simulink model "testALU"  (R2025b)
settings: Solver=VariableStepAuto  StartTime=0.0  StopTime=10.0  RelTol=1e-3
settings Model: Creator=cyber  LastModifiedBy=cyber

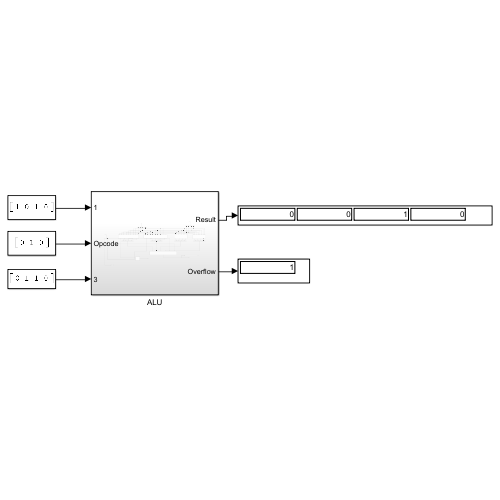
[thumbnail: Simulink's stored preview of the top-level diagram]
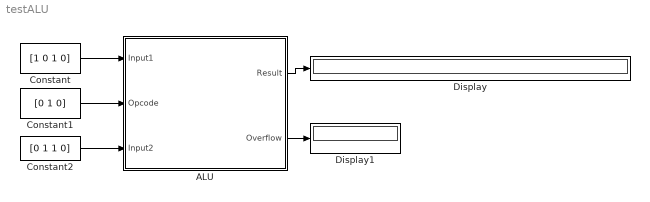
== system testALU ==
  ALU : Subsystem
  Constant : Constant  Value=[1 0 1 0]
  Constant1 : Constant  Value=[0 1 0]
  Constant2 : Constant  Value=[0 1 1 0]
  Display : Display
  Display1 : Display
  wires:
  Constant/1 -> ALU/1(Input1)
  Constant1/1 -> ALU/2(Opcode)
  Constant2/1 -> ALU/3(Input2)
  ALU/1(Result) -> Display/1
  ALU/2(Overflow) -> Display1/1

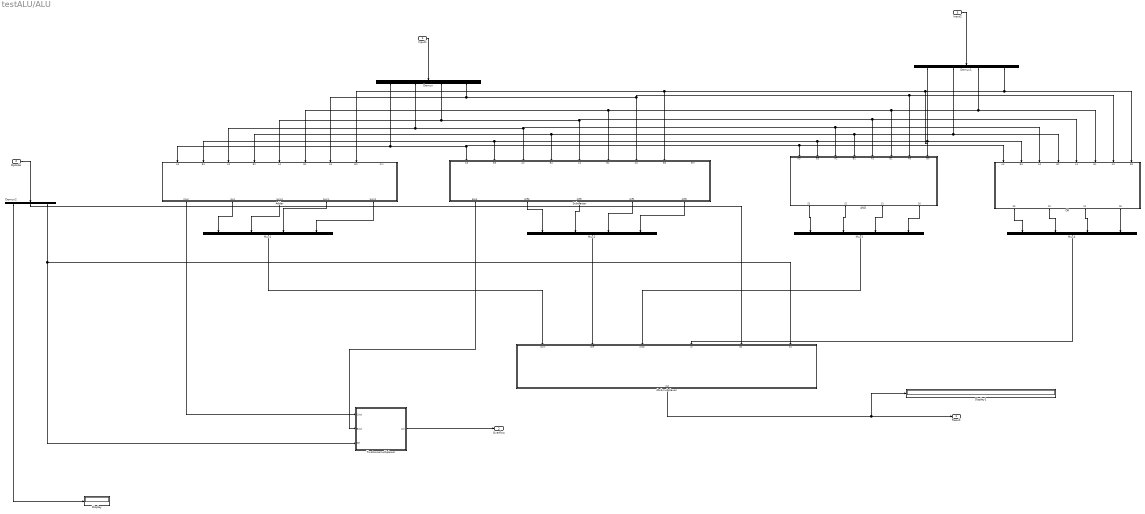
== system testALU/ALU ==
  Input1 : Inport
  Opcode : Inport  Port=2
  Input2 : Inport  Port=3
  4to1multplexer : Subsystem
  AND : Subsystem
  Adder : Subsystem
  Demux : Demux
  Demux1 : Demux
  Demux2 : Demux  Outputs=3
  Display : Display
  Display1 : Display
  Mux{1..4} (4 alike) : Mux
  OR : Subsystem
  Subtractor : Subsystem
  Twotoonemultiplexer : Subsystem
  Result : Outport
  Overflow : Outport  Port=2
  wires:
  Demux2/1 -> Display/1
  Demux1/2 -> OR/4(B2), Adder/4(B2), Subtractor/4(B2), AND/4(B2)
  Mux2/1 -> 4to1multplexer/2(Diff)
  Demux/1 -> OR/1(A3), AND/1(A3), Subtractor/1(A3), Adder/1(A3)
  Adder/2(Sum) -> Mux1/1
  Demux1/4 -> OR/8(B0), AND/8(B0), Adder/8(B0), Subtractor/8(B0)
  Demux/4 -> OR/7(A0), AND/7(A0), Subtractor/7(A0), Adder/7(A0)
  Demux/2 -> OR/3(A2), AND/3(A2), Subtractor/3(A2), Adder/3(A2)
  Demux1/3 -> OR/6(B1), Adder/6(B1), Subtractor/6(B1), AND/6(B1)
  Demux2/3 -> Twotoonemultiplexer/3(Sel), 4to1multplexer/6(S1)
  Demux1/1 -> OR/2(B3), Adder/2(B3), Subtractor/2(B3), AND/2(B3)
  Subtractor/3(Diff2) -> Mux2/2
  Demux/3 -> OR/5(A1), AND/5(A1), Subtractor/5(A1), Adder/5(A1)
  Subtractor/2(Diff3) -> Mux2/1
  Mux4/1 -> 4to1multplexer/4(or)
  Subtractor/1(Bout) -> Twotoonemultiplexer/2(Bout)
  Demux2/2 -> 4to1multplexer/5(S0)
  Subtractor/5(Diff0) -> Mux2/4
  Adder/3(Sum3) -> Mux1/2
  Mux3/1 -> 4to1multplexer/3(AND)
  Adder/4(Sum1) -> Mux1/3
  Adder/1(Cout) -> Twotoonemultiplexer/1(Cout)
  Mux1/1 -> 4to1multplexer/1(Sum)
  Opcode/1 -> Demux2/1
  Twotoonemultiplexer/1(out) -> Overflow/1
  Adder/5(Sum2) -> Mux1/4
  Subtractor/4(Diff1) -> Mux2/3
  4to1multplexer/1(out) -> Display1/1, Result/1
  Input1/1 -> Demux/1
  Input2/1 -> Demux1/1
  AND/1(S3) -> Mux3/1
  AND/2(S2) -> Mux3/2
  AND/3(S1) -> Mux3/3
  AND/4(S0) -> Mux3/4
  OR/1(S3) -> Mux4/1
  OR/2(S2) -> Mux4/2
  OR/3(S1) -> Mux4/3
  OR/4(S0) -> Mux4/4

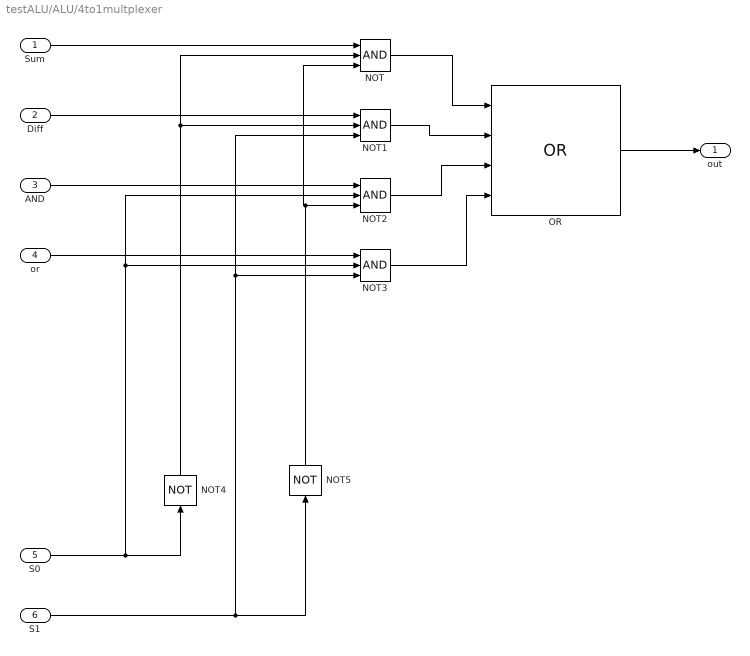
== system testALU/ALU/4to1multplexer ==
  Sum : Inport
  Diff : Inport  Port=2
  AND : Inport  Port=3
  or : Inport  Port=4
  S0 : Inport  Port=5
  S1 : Inport  Port=6
  NOT{,1..3} (4 alike) : Logic  Inputs=3  IconShape=distinctive  AllPortsSameDT=off  OutDataTypeStr=boolean
  NOT4 : Logic  Operator=NOT  IconShape=distinctive  AllPortsSameDT=off  OutDataTypeStr=boolean
  NOT5 : Logic  Operator=NOT  IconShape=distinctive  AllPortsSameDT=off  OutDataTypeStr=boolean
  OR : Logic  Operator=OR  Inputs=4  IconShape=distinctive  AllPortsSameDT=off  OutDataTypeStr=boolean
  out : Outport
  wires:
  NOT4/1 -> NOT/2, NOT1/2
  S1/1 -> NOT1/3, NOT3/3, NOT5/1
  NOT5/1 -> NOT/3, NOT2/3
  NOT1/1 -> OR/2
  S0/1 -> NOT4/1, NOT3/2, NOT2/2
  NOT3/1 -> OR/4
  NOT/1 -> OR/1
  NOT2/1 -> OR/3
  or/1 -> NOT3/1
  Sum/1 -> NOT/1
  AND/1 -> NOT2/1
  Diff/1 -> NOT1/1
  OR/1 -> out/1

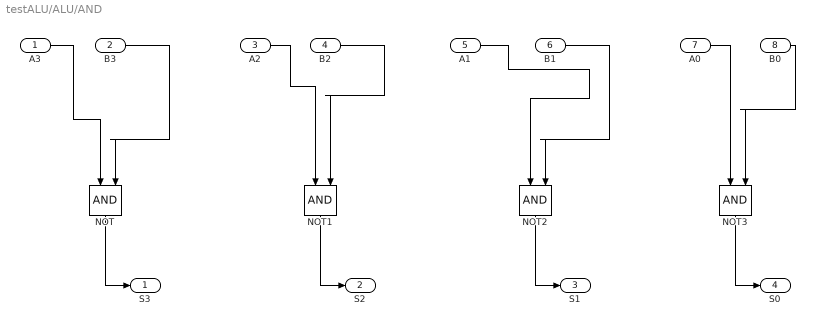
== system testALU/ALU/AND ==
  A3 : Inport
  B3 : Inport  Port=2
  A2 : Inport  Port=3
  B2 : Inport  Port=4
  A1 : Inport  Port=5
  B1 : Inport  Port=6
  A0 : Inport  Port=7
  B0 : Inport  Port=8
  NOT{,1..3} (4 alike) : Logic  IconShape=distinctive  AllPortsSameDT=off  OutDataTypeStr=boolean
  S3 : Outport
  S2 : Outport  Port=2
  S1 : Outport  Port=3
  S0 : Outport  Port=4
  wires:
  B0/1 -> NOT3/2
  NOT/1 -> S3/1
  NOT1/1 -> S2/1
  B1/1 -> NOT2/2
  NOT3/1 -> S0/1
  A3/1 -> NOT/1
  NOT2/1 -> S1/1
  A0/1 -> NOT3/1
  B2/1 -> NOT1/2
  A2/1 -> NOT1/1
  B3/1 -> NOT/2
  A1/1 -> NOT2/1

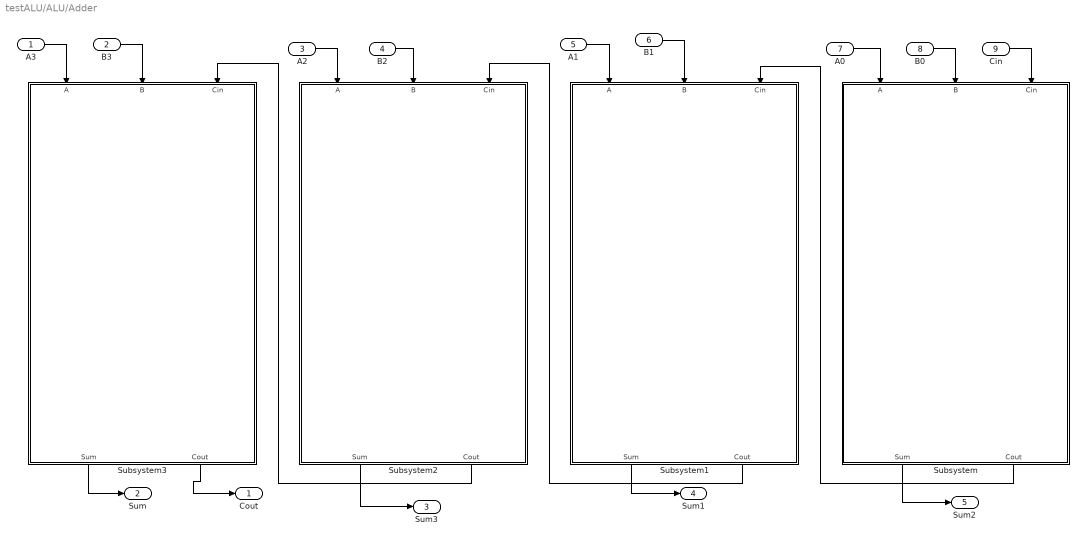
== system testALU/ALU/Adder ==
  A3 : Inport
  B3 : Inport  Port=2
  A2 : Inport  Port=3
  B2 : Inport  Port=4
  A1 : Inport  Port=5
  B1 : Inport  Port=6
  A0 : Inport  Port=7
  B0 : Inport  Port=8
  Cin : Inport  Port=9
  Subsystem : Subsystem
  Subsystem1 : Subsystem
  Subsystem2 : Subsystem
  Subsystem3 : Subsystem
  Cout : Outport
  Sum : Outport  Port=2
  Sum3 : Outport  Port=3
  Sum1 : Outport  Port=4
  Sum2 : Outport  Port=5
  wires:
  Subsystem2/2(Cout) -> Subsystem3/3(Cin)
  B3/1 -> Subsystem3/2(B)
  Subsystem/2(Cout) -> Subsystem1/3(Cin)
  A2/1 -> Subsystem2/1(A)
  A3/1 -> Subsystem3/1(A)
  A1/1 -> Subsystem1/1(A)
  Subsystem/1(Sum) -> Sum2/1
  Subsystem1/2(Cout) -> Subsystem2/3(Cin)
  B1/1 -> Subsystem1/2(B)
  B0/1 -> Subsystem/2(B)
  Subsystem3/1(Sum) -> Sum/1
  B2/1 -> Subsystem2/2(B)
  Subsystem1/1(Sum) -> Sum1/1
  Subsystem2/1(Sum) -> Sum3/1
  Cin/1 -> Subsystem/3(Cin)
  Subsystem3/2(Cout) -> Cout/1
  A0/1 -> Subsystem/1(A)

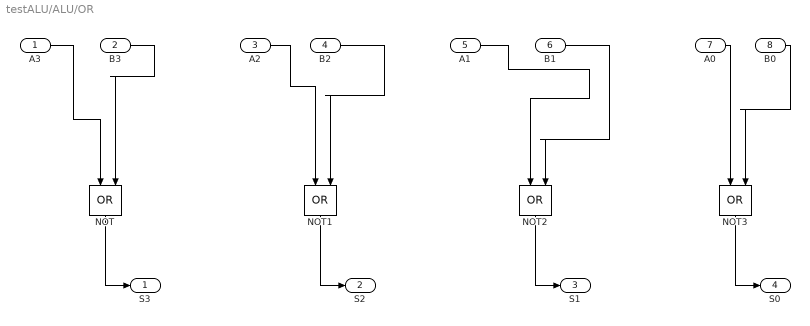
== system testALU/ALU/OR ==
  A3 : Inport
  B3 : Inport  Port=2
  A2 : Inport  Port=3
  B2 : Inport  Port=4
  A1 : Inport  Port=5
  B1 : Inport  Port=6
  A0 : Inport  Port=7
  B0 : Inport  Port=8
  NOT{,1..3} (4 alike) : Logic  Operator=OR  IconShape=distinctive  AllPortsSameDT=off  OutDataTypeStr=boolean
  S3 : Outport
  S2 : Outport  Port=2
  S1 : Outport  Port=3
  S0 : Outport  Port=4
  wires:
  B3/1 -> NOT/2
  B0/1 -> NOT3/2
  A0/1 -> NOT3/1
  NOT3/1 -> S0/1
  A3/1 -> NOT/1
  NOT/1 -> S3/1
  A1/1 -> NOT2/1
  NOT1/1 -> S2/1
  NOT2/1 -> S1/1
  A2/1 -> NOT1/1
  B1/1 -> NOT2/2
  B2/1 -> NOT1/2

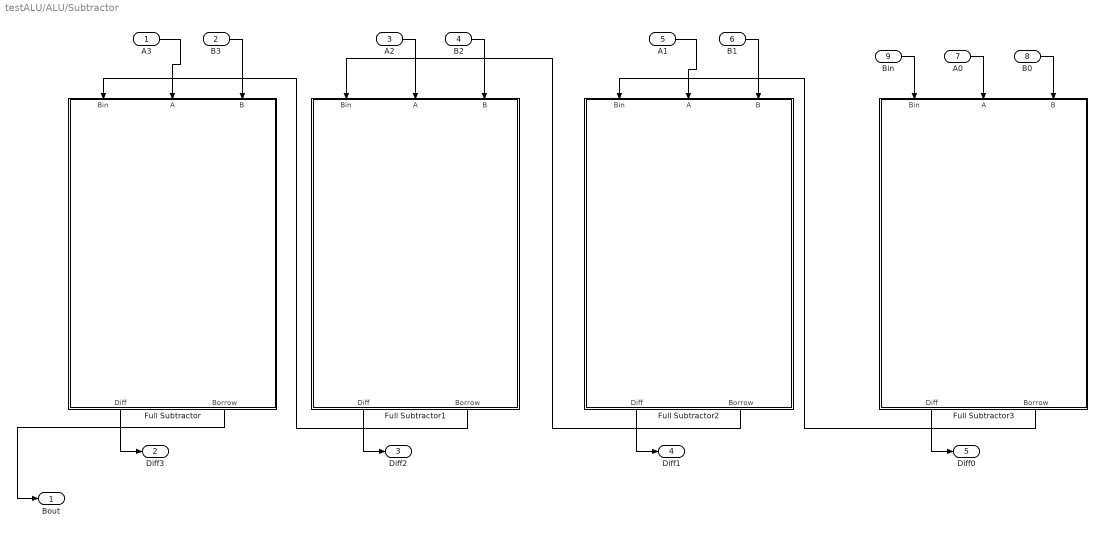
== system testALU/ALU/Subtractor ==
  A3 : Inport
  B3 : Inport  Port=2
  A2 : Inport  Port=3
  B2 : Inport  Port=4
  A1 : Inport  Port=5
  B1 : Inport  Port=6
  A0 : Inport  Port=7
  B0 : Inport  Port=8
  Bin : Inport  Port=9
  Full Subtractor : Subsystem
  Full Subtractor1 : Subsystem
  Full Subtractor2 : Subsystem
  Full Subtractor3 : Subsystem
  Bout : Outport
  Diff3 : Outport  Port=2
  Diff2 : Outport  Port=3
  Diff1 : Outport  Port=4
  Diff0 : Outport  Port=5
  wires:
  Full Subtractor1/1(Diff) -> Diff2/1
  Full Subtractor2/1(Diff) -> Diff1/1
  Full Subtractor3/2(Borrow) -> Full Subtractor2/1(Bin)
  Full Subtractor2/2(Borrow) -> Full Subtractor1/1(Bin)
  Full Subtractor1/2(Borrow) -> Full Subtractor/1(Bin)
  B3/1 -> Full Subtractor/3(B)
  A0/1 -> Full Subtractor3/2(A)
  A2/1 -> Full Subtractor1/2(A)
  Full Subtractor/2(Borrow) -> Bout/1
  Full Subtractor3/1(Diff) -> Diff0/1
  A3/1 -> Full Subtractor/2(A)
  B2/1 -> Full Subtractor1/3(B)
  A1/1 -> Full Subtractor2/2(A)
  B1/1 -> Full Subtractor2/3(B)
  Bin/1 -> Full Subtractor3/1(Bin)
  Full Subtractor/1(Diff) -> Diff3/1
  B0/1 -> Full Subtractor3/3(B)

== system testALU/ALU/Twotoonemultiplexer ==
  Cout : Inport
  Bout : Inport  Port=2
  Sel : Inport  Port=3
  NOT : Logic  IconShape=distinctive  AllPortsSameDT=off  OutDataTypeStr=boolean
  NOT1 : Logic  IconShape=distinctive  AllPortsSameDT=off  OutDataTypeStr=boolean
  NOT2 : Logic  Operator=NOT  IconShape=distinctive  AllPortsSameDT=off  OutDataTypeStr=boolean
  NOT3 : Logic  Operator=OR  IconShape=distinctive  AllPortsSameDT=off  OutDataTypeStr=boolean
  out : Outport
  wires:
  Cout/1 -> NOT/1
  Sel/1 -> NOT1/2, NOT2/1
  NOT1/1 -> NOT3/2
  Bout/1 -> NOT1/1
  NOT2/1 -> NOT/2
  NOT/1 -> NOT3/1
  NOT3/1 -> out/1

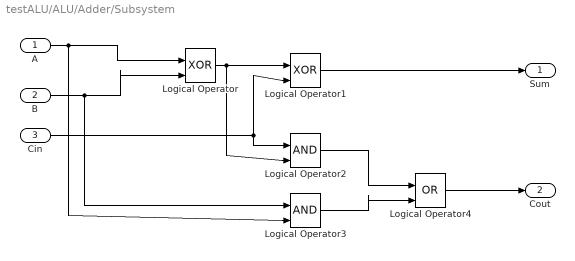
== system testALU/ALU/Adder/Subsystem ==
  A : Inport
  B : Inport  Port=2
  Cin : Inport  Port=3
  Logical Operator : Logic  Operator=XOR  IconShape=distinctive  AllPortsSameDT=off  OutDataTypeStr=boolean
  Logical Operator1 : Logic  Operator=XOR  IconShape=distinctive  AllPortsSameDT=off  OutDataTypeStr=boolean
  Logical Operator2 : Logic  IconShape=distinctive  AllPortsSameDT=off  OutDataTypeStr=boolean
  Logical Operator3 : Logic  IconShape=distinctive  AllPortsSameDT=off  OutDataTypeStr=boolean
  Logical Operator4 : Logic  Operator=OR  IconShape=distinctive  AllPortsSameDT=off  OutDataTypeStr=boolean
  Sum : Outport
  Cout : Outport  Port=2
  wires:
  B/1 -> Logical Operator3/1, Logical Operator/2
  Logical Operator1/1 -> Sum/1
  Logical Operator3/1 -> Logical Operator4/2
  Logical Operator/1 -> Logical Operator2/2, Logical Operator1/1
  Logical Operator4/1 -> Cout/1
  Cin/1 -> Logical Operator2/1, Logical Operator1/2
  Logical Operator2/1 -> Logical Operator4/1
  A/1 -> Logical Operator3/2, Logical Operator/1

== system testALU/ALU/Adder/Subsystem1 ==
  A : Inport
  B : Inport  Port=2
  Cin : Inport  Port=3
  Logical Operator : Logic  Operator=XOR  IconShape=distinctive  AllPortsSameDT=off  OutDataTypeStr=boolean
  Logical Operator1 : Logic  Operator=XOR  IconShape=distinctive  AllPortsSameDT=off  OutDataTypeStr=boolean
  Logical Operator2 : Logic  IconShape=distinctive  AllPortsSameDT=off  OutDataTypeStr=boolean
  Logical Operator3 : Logic  IconShape=distinctive  AllPortsSameDT=off  OutDataTypeStr=boolean
  Logical Operator4 : Logic  Operator=OR  IconShape=distinctive  AllPortsSameDT=off  OutDataTypeStr=boolean
  Sum : Outport
  Cout : Outport  Port=2
  wires:
  B/1 -> Logical Operator3/1, Logical Operator/2
  Logical Operator1/1 -> Sum/1
  Logical Operator3/1 -> Logical Operator4/2
  Logical Operator/1 -> Logical Operator2/2, Logical Operator1/1
  Logical Operator4/1 -> Cout/1
  Cin/1 -> Logical Operator2/1, Logical Operator1/2
  Logical Operator2/1 -> Logical Operator4/1
  A/1 -> Logical Operator3/2, Logical Operator/1

== system testALU/ALU/Adder/Subsystem2 ==
  A : Inport
  B : Inport  Port=2
  Cin : Inport  Port=3
  Logical Operator : Logic  Operator=XOR  IconShape=distinctive  AllPortsSameDT=off  OutDataTypeStr=boolean
  Logical Operator1 : Logic  Operator=XOR  IconShape=distinctive  AllPortsSameDT=off  OutDataTypeStr=boolean
  Logical Operator2 : Logic  IconShape=distinctive  AllPortsSameDT=off  OutDataTypeStr=boolean
  Logical Operator3 : Logic  IconShape=distinctive  AllPortsSameDT=off  OutDataTypeStr=boolean
  Logical Operator4 : Logic  Operator=OR  IconShape=distinctive  AllPortsSameDT=off  OutDataTypeStr=boolean
  Sum : Outport
  Cout : Outport  Port=2
  wires:
  B/1 -> Logical Operator3/1, Logical Operator/2
  Logical Operator1/1 -> Sum/1
  Logical Operator3/1 -> Logical Operator4/2
  Logical Operator/1 -> Logical Operator2/2, Logical Operator1/1
  Logical Operator4/1 -> Cout/1
  Cin/1 -> Logical Operator2/1, Logical Operator1/2
  Logical Operator2/1 -> Logical Operator4/1
  A/1 -> Logical Operator3/2, Logical Operator/1

== system testALU/ALU/Adder/Subsystem3 ==
  A : Inport
  B : Inport  Port=2
  Cin : Inport  Port=3
  Logical Operator : Logic  Operator=XOR  IconShape=distinctive  AllPortsSameDT=off  OutDataTypeStr=boolean
  Logical Operator1 : Logic  Operator=XOR  IconShape=distinctive  AllPortsSameDT=off  OutDataTypeStr=boolean
  Logical Operator2 : Logic  IconShape=distinctive  AllPortsSameDT=off  OutDataTypeStr=boolean
  Logical Operator3 : Logic  IconShape=distinctive  AllPortsSameDT=off  OutDataTypeStr=boolean
  Logical Operator4 : Logic  Operator=OR  IconShape=distinctive  AllPortsSameDT=off  OutDataTypeStr=boolean
  Sum : Outport
  Cout : Outport  Port=2
  wires:
  B/1 -> Logical Operator3/1, Logical Operator/2
  Logical Operator1/1 -> Sum/1
  Logical Operator3/1 -> Logical Operator4/2
  Logical Operator/1 -> Logical Operator2/2, Logical Operator1/1
  Logical Operator4/1 -> Cout/1
  Cin/1 -> Logical Operator2/1, Logical Operator1/2
  Logical Operator2/1 -> Logical Operator4/1
  A/1 -> Logical Operator3/2, Logical Operator/1

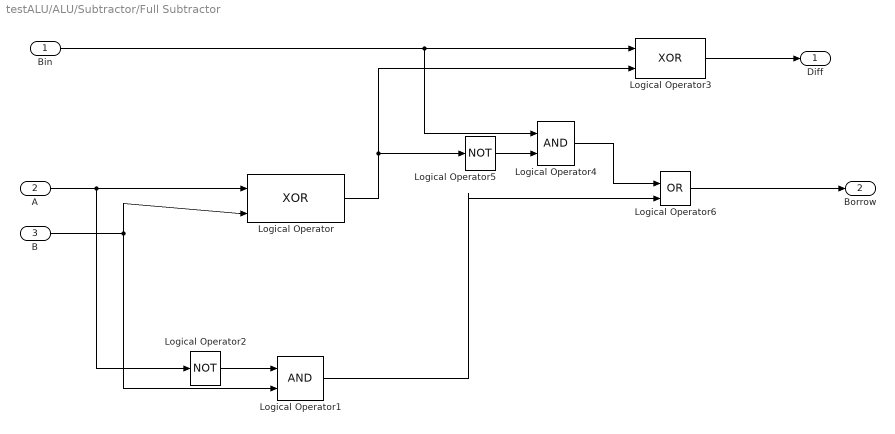
== system testALU/ALU/Subtractor/Full Subtractor ==
  Bin : Inport
  A : Inport  Port=2
  B : Inport  Port=3
  Logical Operator : Logic  Operator=XOR  IconShape=distinctive  AllPortsSameDT=off  OutDataTypeStr=boolean
  Logical Operator1 : Logic  IconShape=distinctive  AllPortsSameDT=off  OutDataTypeStr=boolean
  Logical Operator2 : Logic  Operator=NOT  IconShape=distinctive  AllPortsSameDT=off  OutDataTypeStr=boolean
  Logical Operator3 : Logic  Operator=XOR  IconShape=distinctive  AllPortsSameDT=off  OutDataTypeStr=boolean
  Logical Operator4 : Logic  IconShape=distinctive  AllPortsSameDT=off  OutDataTypeStr=boolean
  Logical Operator5 : Logic  Operator=NOT  IconShape=distinctive  AllPortsSameDT=off  OutDataTypeStr=boolean
  Logical Operator6 : Logic  Operator=OR  IconShape=distinctive  AllPortsSameDT=off  OutDataTypeStr=boolean
  Diff : Outport
  Borrow : Outport  Port=2
  wires:
  Logical Operator/1 -> Logical Operator3/2, Logical Operator5/1
  Logical Operator1/1 -> Logical Operator6/2
  A/1 -> Logical Operator2/1, Logical Operator/1
  Bin/1 -> Logical Operator4/1, Logical Operator3/1
  Logical Operator3/1 -> Diff/1
  B/1 -> Logical Operator/2, Logical Operator1/2
  Logical Operator2/1 -> Logical Operator1/1
  Logical Operator4/1 -> Logical Operator6/1
  Logical Operator5/1 -> Logical Operator4/2
  Logical Operator6/1 -> Borrow/1

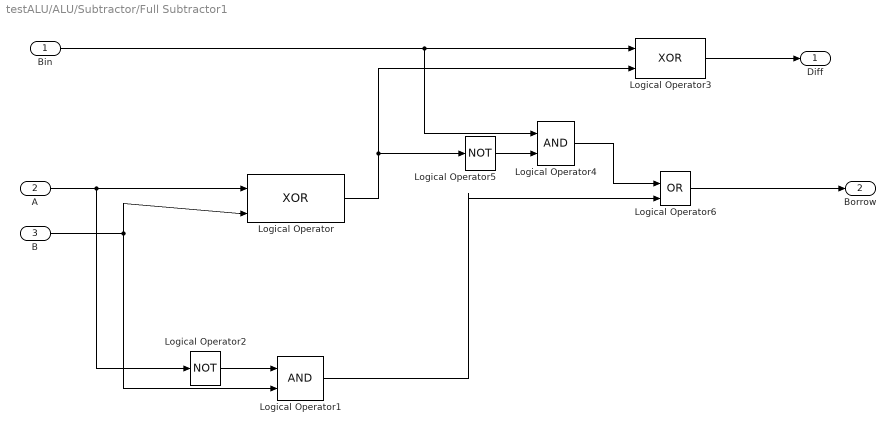
== system testALU/ALU/Subtractor/Full Subtractor1 ==
  Bin : Inport
  A : Inport  Port=2
  B : Inport  Port=3
  Logical Operator : Logic  Operator=XOR  IconShape=distinctive  AllPortsSameDT=off  OutDataTypeStr=boolean
  Logical Operator1 : Logic  IconShape=distinctive  AllPortsSameDT=off  OutDataTypeStr=boolean
  Logical Operator2 : Logic  Operator=NOT  IconShape=distinctive  AllPortsSameDT=off  OutDataTypeStr=boolean
  Logical Operator3 : Logic  Operator=XOR  IconShape=distinctive  AllPortsSameDT=off  OutDataTypeStr=boolean
  Logical Operator4 : Logic  IconShape=distinctive  AllPortsSameDT=off  OutDataTypeStr=boolean
  Logical Operator5 : Logic  Operator=NOT  IconShape=distinctive  AllPortsSameDT=off  OutDataTypeStr=boolean
  Logical Operator6 : Logic  Operator=OR  IconShape=distinctive  AllPortsSameDT=off  OutDataTypeStr=boolean
  Diff : Outport
  Borrow : Outport  Port=2
  wires:
  Logical Operator/1 -> Logical Operator3/2, Logical Operator5/1
  Logical Operator1/1 -> Logical Operator6/2
  A/1 -> Logical Operator2/1, Logical Operator/1
  Bin/1 -> Logical Operator4/1, Logical Operator3/1
  Logical Operator3/1 -> Diff/1
  B/1 -> Logical Operator/2, Logical Operator1/2
  Logical Operator2/1 -> Logical Operator1/1
  Logical Operator4/1 -> Logical Operator6/1
  Logical Operator5/1 -> Logical Operator4/2
  Logical Operator6/1 -> Borrow/1

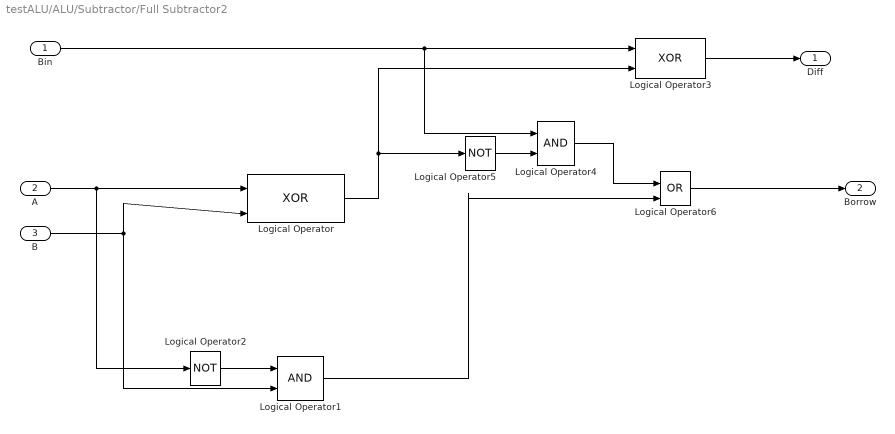
== system testALU/ALU/Subtractor/Full Subtractor2 ==
  Bin : Inport
  A : Inport  Port=2
  B : Inport  Port=3
  Logical Operator : Logic  Operator=XOR  IconShape=distinctive  AllPortsSameDT=off  OutDataTypeStr=boolean
  Logical Operator1 : Logic  IconShape=distinctive  AllPortsSameDT=off  OutDataTypeStr=boolean
  Logical Operator2 : Logic  Operator=NOT  IconShape=distinctive  AllPortsSameDT=off  OutDataTypeStr=boolean
  Logical Operator3 : Logic  Operator=XOR  IconShape=distinctive  AllPortsSameDT=off  OutDataTypeStr=boolean
  Logical Operator4 : Logic  IconShape=distinctive  AllPortsSameDT=off  OutDataTypeStr=boolean
  Logical Operator5 : Logic  Operator=NOT  IconShape=distinctive  AllPortsSameDT=off  OutDataTypeStr=boolean
  Logical Operator6 : Logic  Operator=OR  IconShape=distinctive  AllPortsSameDT=off  OutDataTypeStr=boolean
  Diff : Outport
  Borrow : Outport  Port=2
  wires:
  Logical Operator/1 -> Logical Operator3/2, Logical Operator5/1
  Logical Operator1/1 -> Logical Operator6/2
  A/1 -> Logical Operator2/1, Logical Operator/1
  Bin/1 -> Logical Operator4/1, Logical Operator3/1
  Logical Operator3/1 -> Diff/1
  B/1 -> Logical Operator/2, Logical Operator1/2
  Logical Operator2/1 -> Logical Operator1/1
  Logical Operator4/1 -> Logical Operator6/1
  Logical Operator5/1 -> Logical Operator4/2
  Logical Operator6/1 -> Borrow/1

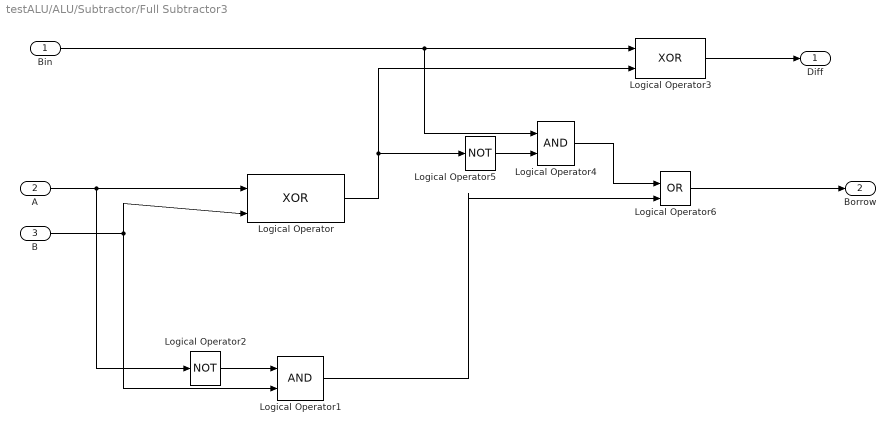
== system testALU/ALU/Subtractor/Full Subtractor3 ==
  Bin : Inport
  A : Inport  Port=2
  B : Inport  Port=3
  Logical Operator : Logic  Operator=XOR  IconShape=distinctive  AllPortsSameDT=off  OutDataTypeStr=boolean
  Logical Operator1 : Logic  IconShape=distinctive  AllPortsSameDT=off  OutDataTypeStr=boolean
  Logical Operator2 : Logic  Operator=NOT  IconShape=distinctive  AllPortsSameDT=off  OutDataTypeStr=boolean
  Logical Operator3 : Logic  Operator=XOR  IconShape=distinctive  AllPortsSameDT=off  OutDataTypeStr=boolean
  Logical Operator4 : Logic  IconShape=distinctive  AllPortsSameDT=off  OutDataTypeStr=boolean
  Logical Operator5 : Logic  Operator=NOT  IconShape=distinctive  AllPortsSameDT=off  OutDataTypeStr=boolean
  Logical Operator6 : Logic  Operator=OR  IconShape=distinctive  AllPortsSameDT=off  OutDataTypeStr=boolean
  Diff : Outport
  Borrow : Outport  Port=2
  wires:
  Logical Operator/1 -> Logical Operator3/2, Logical Operator5/1
  Logical Operator1/1 -> Logical Operator6/2
  A/1 -> Logical Operator2/1, Logical Operator/1
  Bin/1 -> Logical Operator4/1, Logical Operator3/1
  Logical Operator3/1 -> Diff/1
  B/1 -> Logical Operator/2, Logical Operator1/2
  Logical Operator2/1 -> Logical Operator1/1
  Logical Operator4/1 -> Logical Operator6/1
  Logical Operator5/1 -> Logical Operator4/2
  Logical Operator6/1 -> Borrow/1
